simulink model "midterm"  (R2023b)
settings: Solver=VariableStepAuto  StartTime=0.0  StopTime=3  RelTol=1e-3
values from neighbouring files (symbols this model uses):
  a = 1.14    [init.m]
  b = L-a    (= 1.4)    [init.m]
  Caf = 44000*2    (= 88000)    [init.m]
  Car = 47000*2    (= 94000)    [init.m]
  Iz = 2420    [init.m]
  K_r = (m*u_0^2*a-b*(a+b)*Car)/       (m*u_0^2*b-a*(a+b)*Caf)*        Caf/Car    (= 0.217116529413)    [init.m]
  m = 1500    [init.m]
  u_0 = 15    [init.m]
libraries: slpidlib x1
settings Model: Creator=yusufcagriogut  LastModifiedBy=yusufcagriogut

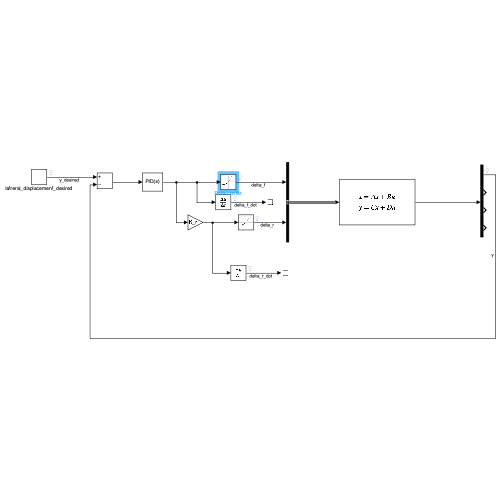
[thumbnail: Simulink's stored preview of the top-level diagram]
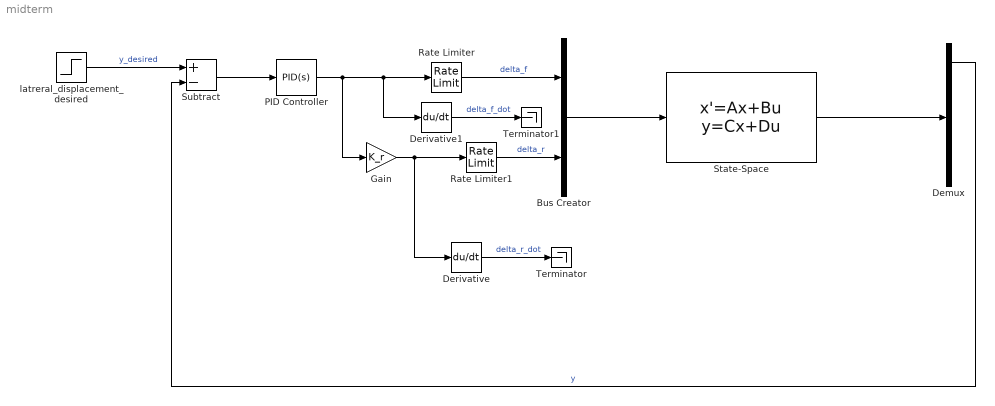
== system midterm ==
  Bus Creator : BusCreator  Inputs=2
  Demux : Demux
  Derivative : Derivative
  Derivative1 : Derivative
  Gain : Gain  Gain=K_r
  PID Controller : slpidlib/PID Controller  Controller=PID  Form=Parallel  TimeDomain=Continuous-time  UseExternalTs=off  SampleTime=-1  IntegratorMethod=Forward Euler  FilterMethod=Forward Euler  ControllerParametersSource=internal  P=2.21563771017107  I=101.071157256416  UseKiTs=off  D=-0.000116820183747656  N=18966.2234649201  UseFilter=on  TunerSelectOption=Transfer Function Based (PID Tuner App)  InitialConditionSource=internal  InitialConditionForIntegrator=0  InitialConditionForFilter=0  DifferentiatorICPrevScaledInput=0  ExternalReset=none  TrackingMode=off  Kt=1  LimitOutput=off  SatLimitsSource=internal  UpperSaturationLimit=inf  LowerSaturationLimit=-inf  LinearizeAsGain=on  AntiWindupMode=none  Kb=1  LimitIntegrator=off  UpperIntegratorSaturationLimit=inf  LowerIntegratorSaturationLimit=-inf  POutMin=[]  POutMax=[]  IOutMin=[]  IOutMax=[]  DOutMin=[]  DOutMax=[]  NOutMin=[]  NOutMax=[]  SumOutMin=[]  SumOutMax=[]  SaturationOutMin=[]  SaturationOutMax=[]  PParamMin=[]  PParamMax=[]  IParamMin=[]  IParamMax=[]  DParamMin=[]  DParamMax=[]  NParamMin=[]  NParamMax=[]  KbParamMin=[]  KbParamMax=[]  KtParamMin=[]  KtParamMax=[]  KbOutMin=[]  KbOutMax=[]  KtOutMin=[]  KtOutMax=[]  IntegratorOutMin=[]  IntegratorOutMax=[]  FilterOutMin=[]  FilterOutMax=[]  SumI1OutMin=[]  SumI1OutMax=[]  SumI2OutMin=[]  SumI2OutMax=[]  SumI3OutMin=[]  SumI3OutMax=[]  SumI4OutMin=[]  SumI4OutMax=[]  SumDOutMin=[]  SumDOutMax=[]  DifferentiatorOutMin=[]  DifferentiatorOutMax=[]  FilterDiffOutCoefMin=[]  FilterDiffOutCoefMax=[]  ReciprocalOutMin=[]  ReciprocalOutMax=[]  SumDenOutMin=[]  SumDenOutMax=[]  SumNumOutMin=[]  SumNumOutMax=[]  DivideOutMin=[]  DivideOutMax=[]  UdiffTsProdOutMin=[]  UdiffTsProdOutMax=[]  NTsProdOutMin=[]  NTsProdOutMax=[]  UintegralTsProdOutMin=[]  UintegralTsProdOutMax=[]  UngainTsProdOutMin=[]  UngainTsProdOutMax=[]  ClampingZeroOutDataTypeStr=Inherit: Inherit via back propagation  ClampingZeroOutMin=[]  ClampingZeroOutMax=[]  FilterDenConstantOutDataTypeStr=Inherit: Inherit via back propagation  FilterDenConstantOutMin=[]  FilterDenConstantOutMax=[]  PCopyOutDataTypeStr=Inherit: Inherit via back propagation  PCopyOutMin=[]  PCopyOutMax=[]  NCopyOutDataTypeStr=Inherit: Inherit via back propagation  NCopyOutMin=[]  NCopyOutMax=[]  IntegratorContinuousStateAttributes=''  IntegratorStateMustResolveToSignalObject=off  IntegratorRTWStateStorageClass=Auto  FilterContinuousStateAttributes=''  FilterStateMustResolveToSignalObject=off  FilterRTWStateStorageClass=Auto  ParallelPVariant=InternalParameters  IdealPVariant=Disabled  IVariant=InternalParameters  DVariant=InternalParameters  IntegratorVariant=Continuous  SatVariant=Disabled  AWVariant=Passthrough  PCopyVariant=Disabled  TRVariant=Disabled  FdbkBlocksVariant=Forward  IdealPFdbkVariant=Disabled  SatFdbkVariant=Disabled  DerivativeFilterVariant=ContFilter  NVariant=InternalParameters  NCopyVariant=Disabled  FilterICVariant=InternalICsFilter  IntegratorICVariant=InternalICs  ExternalResetVariant=Disabled  TRSumVariant=Passthrough  SumFdbkVariant=Disabled  SumVariant=Sum_PID  TsampFilterVariant=InternalTs  TsampNgainVariant=Passthrough  TsampIntegralVariant=Disabled_SignalSpec  ExternalSaturationOutDataTypeStr=Inherit: Same as second input
  Rate Limiter : RateLimiter  RisingSlewLimit=100  FallingSlewLimit=-100  SampleTimeMode=inherited
  Rate Limiter1 : RateLimiter  RisingSlewLimit=100  FallingSlewLimit=-100  SampleTimeMode=inherited
  State-Space : StateSpace  A=[0, 1, u_0, 0; 0, -(Caf+Car)/(m*u_0), 0, (b*Car-a*Caf)/(m*u_0)-u_0; 0, 0, 0, 1; 0, (b*Car-a*Caf)/(Iz*u_0), 0, -(Caf*a^2+Car*b^2)/(Iz*u_0)]  B=[0, 0; Caf/m, Car/m; 0, 0; a*Caf/Iz, -b*Car/Iz]  C=[0, 1, u_0, 0; 0, -(Caf+Car)/(m*u_0), 0, (b*Car-a*Caf)/(m*u_0)-u_0; 0, 0, 0, 1; 0, (b*Car-a*Caf)/(Iz*u_0), 0, -(Caf*a^2+Car*b^2)/(Iz*u_0)]  D=zeros(4,2)  InitialCondition=0
  Subtract : Sum  Inputs=+-
  Terminator : Terminator
  Terminator1 : Terminator
  latreral_displacement_desired : Step  Time=0  SampleTime=0
  wires:
  Bus Creator/1 -> State-Space/1
  State-Space/1 -> Demux/1
  Demux/1 -> Subtract/2  "y"
  Subtract/1 -> PID Controller/1
  latreral_displacement_desired/1 -> Subtract/1  "y_desired"
  PID Controller/1 -> Gain/1, Derivative1/1, Rate Limiter/1
  Gain/1 -> Derivative/1, Rate Limiter1/1
  Derivative/1 -> Terminator/1  "delta_r_dot"
  Derivative1/1 -> Terminator1/1  "delta_f_dot"
  Rate Limiter/1 -> Bus Creator/1  "delta_f"
  Rate Limiter1/1 -> Bus Creator/2  "delta_r"
